simulink model "Lab1_schema"  (R2024a)
settings: Solver=VariableStepAuto  StartTime=0.0  StopTime=10.0  RelTol=1e-3
values from neighbouring files (symbols this model uses):
  Cvp = cpp * rop * Vp    (= 75000)    [Lab1_Badania_script.m]    (also in Lab1_script.m)
  Cvw = cpp * rop * Vw    (= 300000)    [Lab1_Badania_script.m]    (also in Lab1_script.m)
  czas_skoku = 500    [Lab1_Badania_script.m]    (also in Lab1_script.m)
  dPg = 300    [Lab1_Badania_script.m]    (also in Lab1_script.m = 0)
  dTzew = 0    [Lab1_Badania_script.m]    (also in Lab1_script.m = 1)
  K1 = a * Kp    (= 240)    [Lab1_Badania_script.m]    (also in Lab1_script.m)
  Kd = (Kp * (TwewN - TpN)) / (TpN - TzewN)    (= 11.4285714286)    [Lab1_Badania_script.m]    (also in Lab1_script.m)
  Kp = PgN / ((a + 1) * TwewN - a * TzewN - TpN)    (= 80)    [Lab1_Badania_script.m]    (also in Lab1_script.m)
  Pg0 = tab_Pg(i)    [Lab1_Badania_script.m]    (also in Lab1_script.m = 10000)
  Tp0 = (Kp * Twew0 + Kd * Tzew0) / (Kp + Kd)    (= 15)    [Lab1_Badania_script.m]    (also in Lab1_script.m)
  Twew0 = (Pg0 * (Kp + Kd)) / (Kp * (a * Kp + (a + 1) * Kd)) + Tzew0    (= 20)    [Lab1_Badania_script.m]    (also in Lab1_script.m)
  Tzew0 = tab_Tzew(i)    [Lab1_Badania_script.m]    (also in Lab1_script.m = -20)
settings Model: Creator=macie  LastModifiedBy=macie

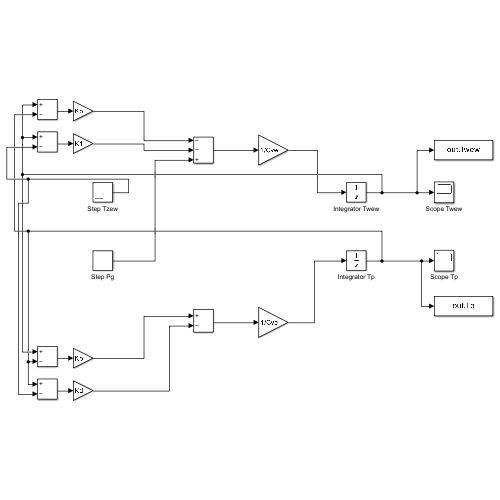
[thumbnail: Simulink's stored preview of the top-level diagram]
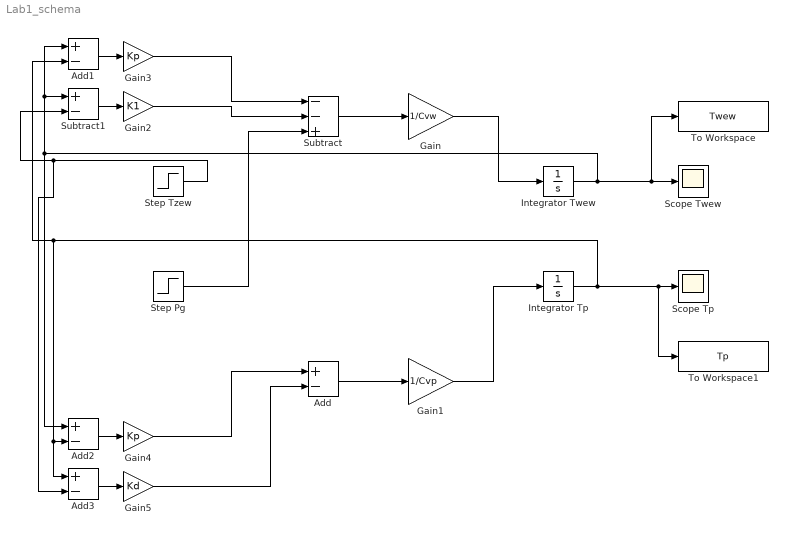
== system Lab1_schema ==
  Add{,1..3} (4 alike) : Sum  Inputs=+-
  Gain : Gain  Gain=1/Cvw
  Gain1 : Gain  Gain=1/Cvp
  Gain2 : Gain  Gain=K1
  Gain3 : Gain  Gain=Kp
  Gain4 : Gain  Gain=Kp
  Gain5 : Gain  Gain=Kd
  Integrator Tp : Integrator  InitialCondition=Tp0
  Integrator Twew : Integrator  InitialCondition=Twew0
  Scope Tp : Scope
  Scope Twew : Scope
  Step Pg : Step  Time=czas_skoku  Before=Pg0  After=Pg0 + dPg  SampleTime=0
  Step Tzew : Step  Time=czas_skoku  Before=Tzew0  After=Tzew0 + dTzew  SampleTime=0  VectorParams1D=off
  Subtract : Sum  Inputs=--+
  Subtract1 : Sum  Inputs=+-
  To Workspace : ToWorkspace  VariableName=Twew  SampleTime=-1
  To Workspace1 : ToWorkspace  VariableName=Tp  SampleTime=-1
  wires:
  Subtract/1 -> Gain/1
  Add/1 -> Gain1/1
  Step Pg/1 -> Subtract/3
  Integrator Twew/1 -> To Workspace/1, Scope Twew/1, Add2/1, Add1/1, Subtract1/1
  Step Tzew/1 -> Add3/2, Subtract1/2
  Subtract1/1 -> Gain2/1
  Gain2/1 -> Subtract/2
  Integrator Tp/1 -> To Workspace1/1, Scope Tp/1, Add3/1, Add2/2, Add1/2
  Add1/1 -> Gain3/1
  Gain3/1 -> Subtract/1
  Gain/1 -> Integrator Twew/1
  Add2/1 -> Gain4/1
  Add3/1 -> Gain5/1
  Gain4/1 -> Add/1
  Gain5/1 -> Add/2
  Gain1/1 -> Integrator Tp/1
